simulink model "ej3"  (R2013a)
settings: Solver=ode45  StartTime=0.0  StopTime=10.0  RelTol=1e-3
settings Model: Creator=nazaretrogue  LastModifiedBy=nazaretrogue

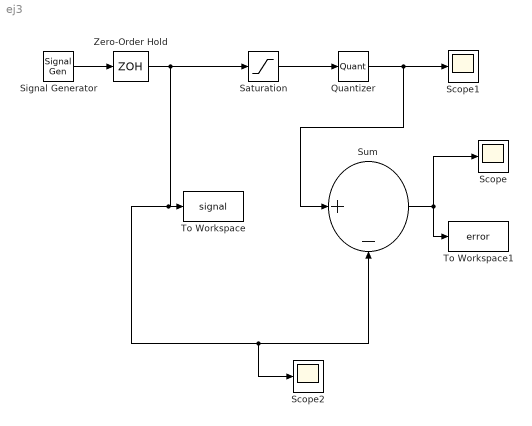
== system ej3 ==
  Quantizer : Quantizer  QuantizationInterval=2/16
  Saturation : Saturate  UpperLimit=1  LowerLimit=-1
  Scope : Scope
  Scope1 : Scope
  Scope2 : Scope
      settings: SaveName=ScopeData2
  Signal Generator : SignalGenerator
  Sum : Sum  Inputs=|+-
  To Workspace : ToWorkspace  VariableName=signal  SampleTime=-1  SaveFormat=Timeseries
  To Workspace1 : ToWorkspace  VariableName=error  SampleTime=-1  SaveFormat=Timeseries
  Zero-Order Hold : ZeroOrderHold  SampleTime=0.02
  wires:
  Signal Generator/1 -> Zero-Order Hold/1
  Zero-Order Hold/1 -> Saturation/1, Scope2/1, Sum/2, To Workspace/1
  Saturation/1 -> Quantizer/1
  Quantizer/1 -> Sum/1, Scope1/1
  Sum/1 -> Scope/1, To Workspace1/1
